simulink model "modelo_quarto_veiculo"  (R2025a)
settings: Solver=VariableStepAuto  StartTime=0.0  StopTime=10.0  RelTol=1e-3
undefined symbols (not defined in the file): cs, ks, kt, ms_q, mus_q
settings Model: Creator=Anderson  LastModifiedBy=Anderson

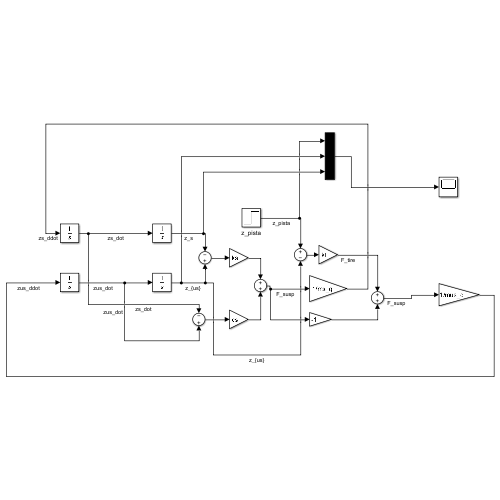
[thumbnail: Simulink's stored preview of the top-level diagram]
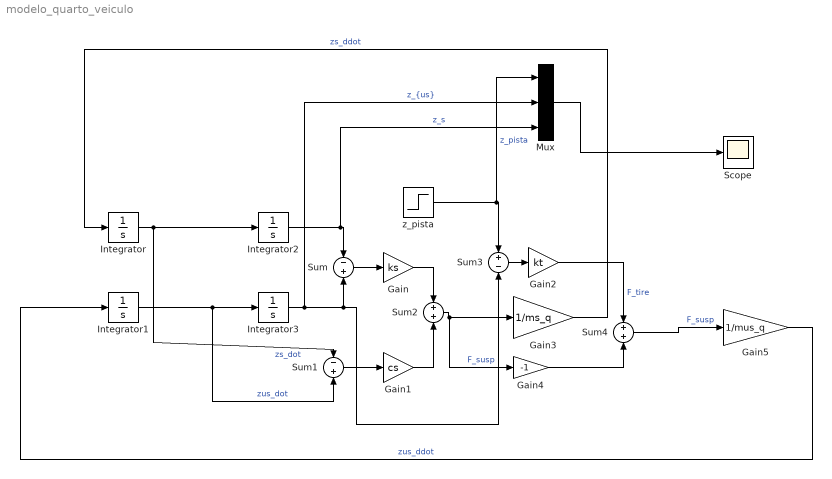
== system modelo_quarto_veiculo ==
  Gain : Gain  Gain=ks
  Gain1 : Gain  Gain=cs
  Gain2 : Gain  Gain=kt
  Gain3 : Gain  Gain=1/ms_q
  Gain4 : Gain  Gain=-1
  Gain5 : Gain  Gain=1/mus_q
  Integrator{,1..3} (4 alike) : Integrator
  Mux : Mux  Inputs=3
  Scope : Scope
      settings: ActiveDisplayYMinimum=-0.018000867451052643  ActiveDisplayYMaximum=0.16200780705947382
  Sum : Sum  Inputs=-+
  Sum1 : Sum  Inputs=-+
  Sum2 : Sum
  Sum3 : Sum  Inputs=+-
  Sum4 : Sum
  z_pista : Step  After=0.1  SampleTime=0
  wires:
  Integrator/1 -> Integrator2/1, Sum1/1  "zs_dot"
  Gain3/1 -> Integrator/1  "zs_ddot"
  Integrator2/1 -> Mux/3, Sum/1  "z_s"
  Gain5/1 -> Integrator1/1  "zus_ddot"
  Integrator1/1 -> Integrator3/1, Sum1/2  "zus_dot"
  Integrator3/1 -> Mux/2, Sum3/2, Sum/2  "z_{us}"
  Sum/1 -> Gain/1
  Sum1/1 -> Gain1/1
  Gain/1 -> Sum2/1
  Gain1/1 -> Sum2/2
  Sum2/1 -> Gain4/1, Gain3/1  "F_susp"
  z_pista/1 -> Mux/1, Sum3/1  "z_pista"
  Sum3/1 -> Gain2/1
  Gain2/1 -> Sum4/1  "F_tire"
  Gain4/1 -> Sum4/2
  Sum4/1 -> Gain5/1  "F_susp"
  Mux/1 -> Scope/1
